simulink model "PID_pitch_test"  (R2024a)
settings: Solver=VariableStepAuto  StartTime=0.0  StopTime=1  RelTol=1e-3
libraries: aerolibconvert2 x1, slpidlib x1, aerolibanimutils x1, simulink_extras x1, uavutilslib x1
settings Model: PacingRate=2  Creator=jliu3  LastModifiedBy=jliu3

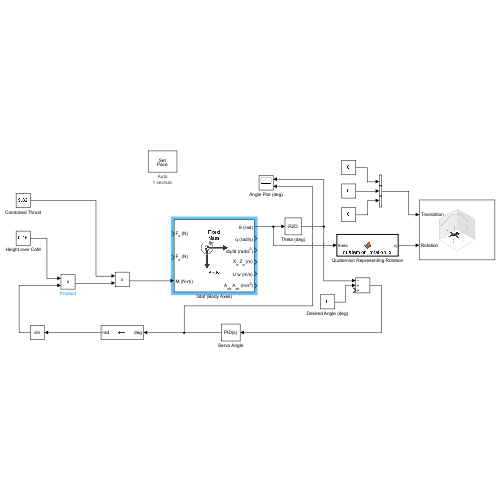
[thumbnail: Simulink's stored preview of the top-level diagram]
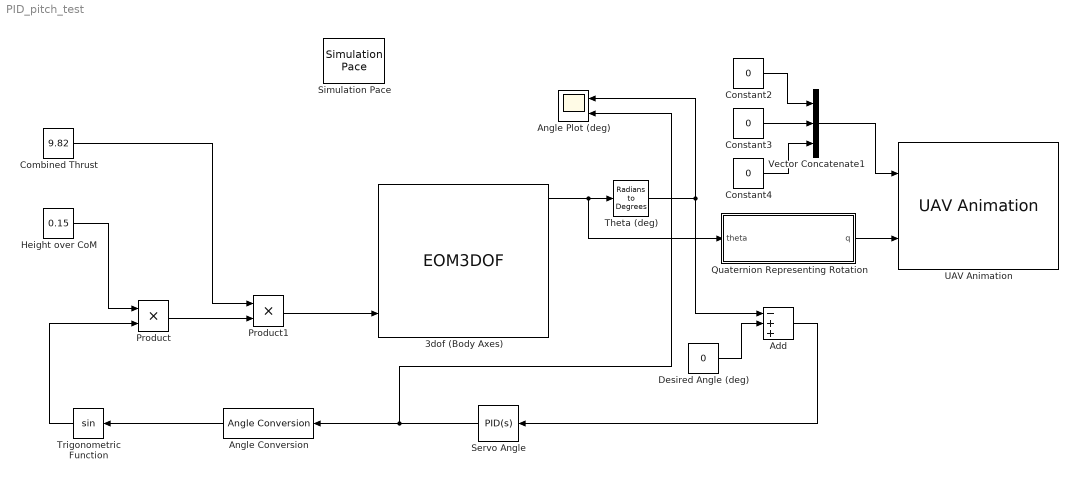
== system PID_pitch_test ==
  3dof (Body Axes) : EOM3DOF  v_ini=0  theta_ini=0.0872665  mass=1.2  Iyy=0.0043
  Add : Sum  Inputs=-++
  Angle Conversion : aerolibconvert2/Angle Conversion  IU=deg  OU=rad
  Angle Plot (deg) : Scope  NumInputPorts=2
  Combined Thrust : Constant  Value=9.82
  Constant2 : Constant  Value=0
  Constant3 : Constant  Value=0
  Constant4 : Constant  Value=0
  Desired Angle (deg) : Constant  Value=0
  "Height over CoM " : Constant  Value=0.15
  Product : Product
  Product1 : Product
  Quaternion Representing Rotation : MATLAB Function  TreatAsAtomicUnit=on
  Servo Angle : slpidlib/PID Controller  Controller=PID  Form=Parallel  TimeDomain=Continuous-time  UseExternalTs=off  SampleTime=-1  IntegratorMethod=Forward Euler  FilterMethod=Forward Euler  ControllerParametersSource=internal  P=0.8  I=0  UseKiTs=off  D=0.2  UseExternalDerivativeSource=off  N=100  UseFilter=on  TunerSelectOption=Transfer Function Based (PID Tuner App)  InitialConditionSource=internal  InitialConditionForIntegrator=0  InitialConditionForFilter=0  DifferentiatorICPrevScaledInput=0  ExternalReset=none  TrackingMode=off  Kt=1  LimitOutput=off  SatLimitsSource=internal  UpperSaturationLimit=inf  LowerSaturationLimit=-inf  LinearizeAsGain=on  AntiWindupMode=none  Kb=1  LimitIntegrator=off  UpperIntegratorSaturationLimit=inf  LowerIntegratorSaturationLimit=-inf  POutMin=[]  POutMax=[]  IOutMin=[]  IOutMax=[]  DOutMin=[]  DOutMax=[]  NOutMin=[]  NOutMax=[]  SumOutMin=[]  SumOutMax=[]  SaturationOutMin=[]  SaturationOutMax=[]  PParamMin=[]  PParamMax=[]  IParamMin=[]  IParamMax=[]  DParamMin=[]  DParamMax=[]  NParamMin=[]  NParamMax=[]  KbParamMin=[]  KbParamMax=[]  KtParamMin=[]  KtParamMax=[]  KbOutMin=[]  KbOutMax=[]  KtOutMin=[]  KtOutMax=[]  IntegratorOutMin=[]  IntegratorOutMax=[]  FilterOutMin=[]  FilterOutMax=[]  SumI1OutMin=[]  SumI1OutMax=[]  SumI2OutMin=[]  SumI2OutMax=[]  SumI3OutMin=[]  SumI3OutMax=[]  SumI4OutMin=[]  SumI4OutMax=[]  SumDOutMin=[]  SumDOutMax=[]  DifferentiatorOutMin=[]  DifferentiatorOutMax=[]  FilterDiffOutCoefMin=[]  FilterDiffOutCoefMax=[]  ReciprocalOutMin=[]  ReciprocalOutMax=[]  SumDenOutMin=[]  SumDenOutMax=[]  SumNumOutMin=[]  SumNumOutMax=[]  DivideOutMin=[]  DivideOutMax=[]  UdiffTsProdOutMin=[]  UdiffTsProdOutMax=[]  NTsProdOutMin=[]  NTsProdOutMax=[]  UintegralTsProdOutMin=[]  UintegralTsProdOutMax=[]  UngainTsProdOutMin=[]  UngainTsProdOutMax=[]  ClampingZeroOutDataTypeStr=Inherit: Inherit via back propagation  ClampingZeroOutMin=[]  ClampingZeroOutMax=[]  FilterDenConstantOutDataTypeStr=Inherit: Inherit via back propagation  FilterDenConstantOutMin=[]  FilterDenConstantOutMax=[]  PCopyOutDataTypeStr=Inherit: Inherit via back propagation  PCopyOutMin=[]  PCopyOutMax=[]  NCopyOutDataTypeStr=Inherit: Inherit via back propagation  NCopyOutMin=[]  NCopyOutMax=[]  IntegratorContinuousStateAttributes=''  IntegratorStateMustResolveToSignalObject=off  IntegratorRTWStateStorageClass=Auto  FilterContinuousStateAttributes=''  FilterStateMustResolveToSignalObject=off  FilterRTWStateStorageClass=Auto  ParallelPVariant=InternalParameters  IdealPVariant=Disabled  IVariant=InternalParameters  DVariant=InternalParameters  IntegratorVariant=Continuous  SatVariant=Disabled  AWVariant=Passthrough  PCopyVariant=Disabled  TRVariant=Disabled  FdbkBlocksVariant=Forward  IdealPFdbkVariant=Disabled  SatFdbkVariant=Disabled  DerivativeFilterVariant=ContFilter  NVariant=InternalParameters  NCopyVariant=Disabled  FilterICVariant=InternalICsFilter  IntegratorICVariant=InternalICs  ExternalResetVariant=Disabled  TRSumVariant=Passthrough  SumFdbkVariant=Disabled  SumVariant=Sum_PID  TsampFilterVariant=InternalTs  TsampNgainVariant=Passthrough  TsampIntegralVariant=Disabled_SignalSpec  ExternalSaturationOutDataTypeStr=Inherit: Same as second input  DerivativeSourceVariant=ErrorSignal
  Simulation Pace : aerolibanimutils/Simulation Pace  SimulationPace=1  SleepMode=Auto  OutputPaceError=off  SampleTime=1/30
  Theta (deg) : simulink_extras/Transformations/Radians to Degrees
  Trigonometric Function : Trigonometry
  UAV Animation : uavutilslib/UAV Animation  UAVType=FixedWing  UAVSize=2.5  InertialZDirection=Down  SampleTime=-1
  Vector Concatenate1 : Concatenate  NumInputs=3
  wires:
  Theta (deg)/1 -> Add/1, Angle Plot (deg)/1
  Product1/1 -> 3dof (Body Axes)/3
  3dof (Body Axes)/1 -> Quaternion Representing Rotation/1(theta), Theta (deg)/1
  Servo Angle/1 -> Angle Plot (deg)/2, Angle Conversion/1
  Add/1 -> Servo Angle/1
  Quaternion Representing Rotation/1(q) -> UAV Animation/2
  Constant2/1 -> Vector Concatenate1/1
  Constant3/1 -> Vector Concatenate1/2
  Constant4/1 -> Vector Concatenate1/3
  Vector Concatenate1/1 -> UAV Animation/1
  Desired Angle (deg)/1 -> Add/2
  "Height over CoM "/1 -> Product/1
  Combined Thrust/1 -> Product1/1
  Angle Conversion/1 -> Trigonometric Function/1
  Trigonometric Function/1 -> Product/2
  Product/1 -> Product1/2

== matlab function PID_pitch_test/Quaternion Representing Rotation ==
  data: theta input; q output
function q = quaternion_rotation_x(theta)
    % create a quaternion representing roll along the x axis from an input
    % angle in radians
    q0 = cos(theta / 2);
    q1 = 0;
    q2 = sin(theta / 2);
    q3 = 0;
    q = [q0 q1 q2 q3];
